simulink model "Commande_TD_EE2"  (R2015a)
settings: Solver=ode45  StartTime=0.0  StopTime=30  RelTol=1e-3
values from neighbouring files (symbols this model uses):
  ftRef = CommTD.ft(1)    [CommandeEE2.m]    (also in CommandeEE2_RetourIntTD.m = CommTD_integral.ft(1))
  ftVs = CommTD.ft(2)    [CommandeEE2.m]    (also in CommandeEE2_RetourIntTD.m = CommTD_integral.ft(2))
  Te = 0.052    [CommandeEE2.m]    (also in CommandeEE2_RetourIntTD.m = 0.026)
undefined symbols (not defined in the file or in its folder): CommTD, EE0, EE1, EE2
settings Model: Creator=David  LastModifiedBy=David

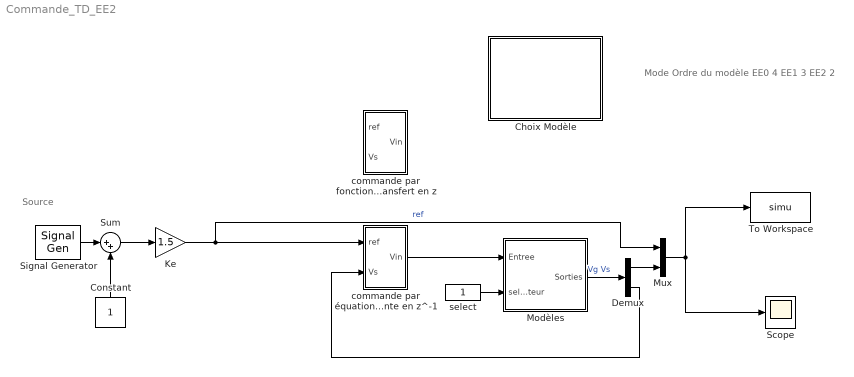
== system Commande_TD_EE2 ==
  note: Mode
      | Ordre du modèle
      |
      | EE0
      | 4
      |
      | EE1
      | 3
      |
      | EE2
      | 2
  note: Source
  Choix Modèle : Subsystem  DialogController=hmiCreateDDGDialog  IsWebBlock=on  mask(MathWorksWebBlock){webBlockId=ad2885e4-e515-47fa-ace6-5d2fe9143339, webBlockType=discreteknob, ShowInLibBrowser=on, ShowInitialText=on, HMISrcModelName=Commande_TD_EE2}
      mask prompts: webBlockId "WebBlock Id"; webBlockType "WebBlock Type"; HMISrcModelName "Source Model"
      mask Help: helpview([docroot '/mapfiles/simulink.map'], 'hmi_rotary_switch')
      mask Display:
      | model = bdroot(gcb);
      | if strcmp(get_param(model,'BlockDiagramType'), 'library')
      |     image([(matlabroot) '/toolbox/simulink/hmi/icons/DiscreteKnob.png']);
      | end
  Constant : Constant
  Demux : Demux  Outputs=2
  Ke : Gain  Gain=1.5  SaturateOnIntegerOverflow=on  OutDataTypeStr=Inherit: Same as input  ParamDataTypeStr=Inherit: Same as input
  Modèles : Subsystem
  Mux : Mux  Inputs=2
  Scope : Scope
      settings: YMin=-0.25  YMax=3.25  SaveName=ScopeData3
  Signal Generator : SignalGenerator  WaveForm=square  Frequency=.1
  Sum : Sum  Inputs=|++  SaturateOnIntegerOverflow=on  InputSameDT=on  OutDataTypeStr=Inherit: Same as first input
  To Workspace : ToWorkspace  VariableName=simu  SaveFormat=Structure With Time  SampleTime=-1
  commande par fonctions de transfert en z : Subsystem
  commande par équation réccurente en z^-1 : Subsystem
  select : Constant
  wires:
  Sum/1 -> Ke/1
  Signal Generator/1 -> Sum/1
  Constant/1 -> Sum/2
  Ke/1 -> commande par équation réccurente en z^-1/1(ref), Mux/1  "ref"
  Mux/1 -> Scope/1, To Workspace/1
  commande par équation réccurente en z^-1/1(Vin) -> Modèles/1(Entree)
  Modèles/1(Sorties) -> Demux/1  "Vg Vs"
  select/1 -> Modèles/2(selecteur)
  Demux/1 -> Mux/2
  Demux/2 -> commande par équation réccurente en z^-1/2(Vs)

== system Commande_TD_EE2/Choix Modèle ==

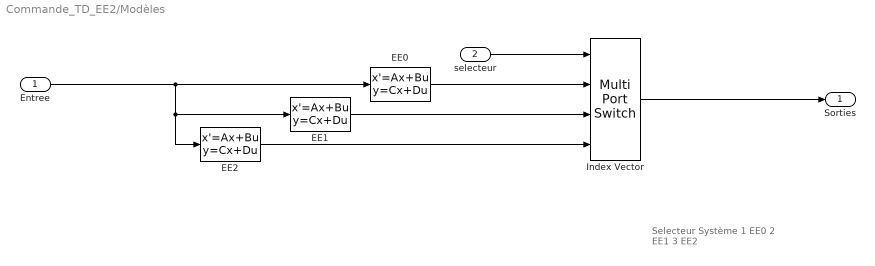
== system Commande_TD_EE2/Modèles ==
  note: Selecteur
      | Système
      |
      | 1
      | EE0
      |
      | 2
      | EE1
      |
      | 3
      | EE2
  Entree : Inport
  selecteur : Inport  Port=2
  EE0 : StateSpace  A=EE0.ee.a  B=EE0.ee.b  C=EE0.ee.c  D=EE0.ee.d  X0=0
  EE1 : StateSpace  A=EE1.ee.a  B=EE1.ee.b  C=EE1.ee.c  D=EE1.ee.d  X0=0
  "EE2 " : StateSpace  A=EE2.ee.a  B=EE2.ee.b  C=EE2.ee.c  D=EE2.ee.d  X0=0
  Index Vector : MultiPortSwitch
  Sorties : Outport
  wires:
  Index Vector/1 -> Sorties/1
  Entree/1 -> "EE2 "/1, EE1/1, EE0/1
  selecteur/1 -> Index Vector/1
  EE0/1 -> Index Vector/2
  EE1/1 -> Index Vector/3
  "EE2 "/1 -> Index Vector/4

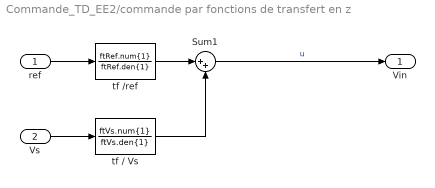
== system Commande_TD_EE2/commande par fonctions de transfert en z ==
  ref : Inport
  Vs : Inport  Port=2
  Sum1 : Sum  Inputs=|++
  tf / Vs : DiscreteTransferFcn  Numerator=ftVs.num{1}  Denominator=ftVs.den{1}  SampleTime=Te
  tf /ref : DiscreteTransferFcn  Numerator=ftRef.num{1}  Denominator=ftRef.den{1}  SampleTime=Te
  Vin : Outport
  wires:
  ref/1 -> tf /ref/1
  tf /ref/1 -> Sum1/1
  Vs/1 -> tf / Vs/1
  tf / Vs/1 -> Sum1/2
  Sum1/1 -> Vin/1  "u"

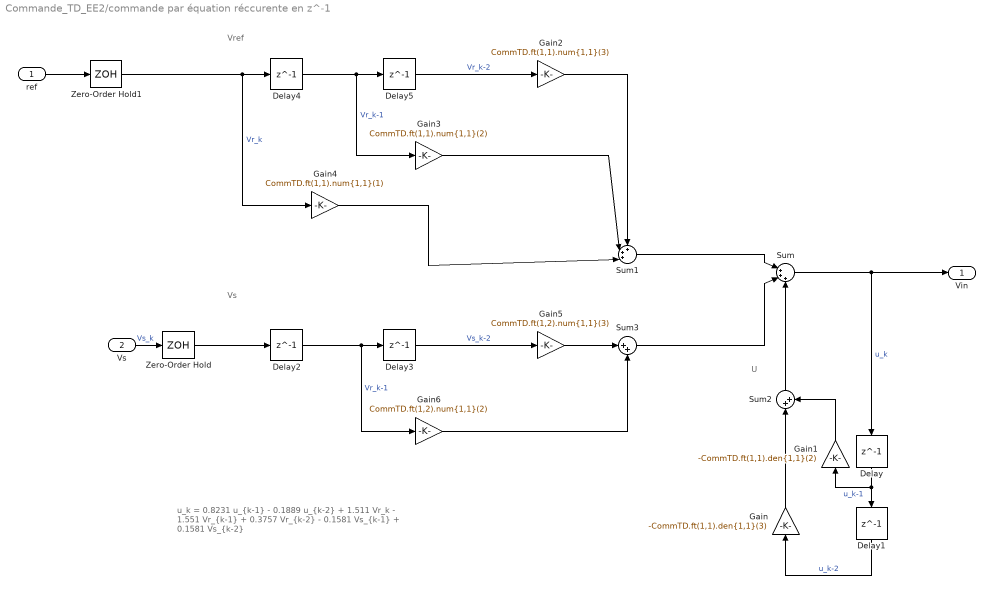
== system Commande_TD_EE2/commande par équation réccurente en z^-1 ==
  note: Vs
  note: Vref
  note: U
  note: u_k = 0.8231 u_{k-1} - 0.1889 u_{k-2}
      | + 1.511 Vr_k - 1.551 Vr_{k-1} + 0.3757 Vr_{k-2}
      | - 0.1581 Vs_{k-1} + 0.1581 Vs_{k-2}
  ref : Inport
  Vs : Inport  Port=2
  Delay{,1..5} (6 alike) : Delay  DelayLength=1  InitialCondition=0  SampleTime=Te
  Gain : Gain  Gain=-CommTD.ft(1,1).den{1,1}(3)
  Gain1 : Gain  Gain=-CommTD.ft(1,1).den{1,1}(2)
  Gain2 : Gain  Gain=CommTD.ft(1,1).num{1,1}(3)
  Gain3 : Gain  Gain=CommTD.ft(1,1).num{1,1}(2)
  Gain4 : Gain  Gain=CommTD.ft(1,1).num{1,1}(1)
  Gain5 : Gain  Gain=CommTD.ft(1,2).num{1,1}(3)
  Gain6 : Gain  Gain=CommTD.ft(1,2).num{1,1}(2)
  Sum : Sum  Inputs=|+++
  Sum1 : Sum  Inputs=+++|
  Sum2 : Sum  Inputs=|++
  Sum3 : Sum  Inputs=|++
  Zero-Order Hold : ZeroOrderHold  SampleTime=Te
  Zero-Order Hold1 : ZeroOrderHold  SampleTime=Te
  Vin : Outport
  wires:
  Vs/1 -> Zero-Order Hold/1  "Vs_k"
  Sum/1 -> Vin/1, Delay/1  "u_k"
  Sum1/1 -> Sum/1
  Delay/1 -> Gain1/1, Delay1/1  "u_k-1"
  Delay1/1 -> Gain/1  "u_k-2"
  Sum2/1 -> Sum/3
  Gain/1 -> Sum2/1
  Gain1/1 -> Sum2/2
  Delay3/1 -> Gain5/1  "Vs_k-2"
  ref/1 -> Zero-Order Hold1/1
  Delay4/1 -> Gain3/1, Delay5/1  "Vr_k-1"
  Delay5/1 -> Gain2/1  "Vr_k-2"
  Gain2/1 -> Sum1/1
  Gain3/1 -> Sum1/2
  Gain4/1 -> Sum1/3
  Sum3/1 -> Sum/2
  Delay2/1 -> Gain6/1, Delay3/1  "Vr_k-1"
  Gain5/1 -> Sum3/1
  Gain6/1 -> Sum3/2
  Zero-Order Hold/1 -> Delay2/1
  Zero-Order Hold1/1 -> Gain4/1, Delay4/1  "Vr_k"
